simulink model "iiwa_IK_FABRIK_ROS (bkp)"  (R2016b)
settings: Solver=FixedStepAuto  StartTime=0.0  StopTime=inf  FixedStep=0.05  RelTol=1e-3
model workspace (MAT data in the model file):
  SL_ROS_VariableLengthArrays_MaxSizes : struct (value not decoded)
libraries: robotlib x7
(part 2 of 2)

== matlab function iiwa_IK_FABRIK_ROS (bkp)/IK/ik_solver ==
  data: Qs output; js_cur_msg input; T input; Qf output; Q2 output; Q3 output; traj_mode output; x_err output; y_err output; z_err output; alpha_err output; betta_err output; gamma_err output; tr_mode input; out_of_trj input boolean; T_ output; R output
% Based on transformation between /iiwa_base_link and /target_frame from tf
% as on error IK problem is solved and corresponding joint angles 
% changes is sent to arm_state topic

function [Qs, Qf, Q2, Q3, traj_mode, x_err, y_err, z_err, alpha_err,... 
          betta_err, gamma_err, T_, R] = fcn(js_cur_msg, T, tr_mode, out_of_trj)
      
persistent points;
if isempty(points)
    points = zeros(7,3);
    
end

persistent on_traj;
if isempty(on_traj)
    on_traj = true;
end

persistent out_of_;
if isempty(out_of_)
    out_of_ = true;
end

persistent seq;
if isempty(seq)
    seq = 0;
end

persistent x;
if isempty(x)
    x = 0;
end

persistent y;
if isempty(y)
    y = 0;
end

persistent z;
if isempty(z)
    z = 0.1;
end

persistent q;
if isempty(q)
    q = [1, 0, 0, 0];
end

T_ = T;

d01 = 0.36;
d23 = 0.42;
d45 = 0.4;
d67 = 0.126;

th1 = js_cur_msg.Position(1);
th2 = js_cur_msg.Position(2);
th3 = js_cur_msg.Position(3);
th4 = js_cur_msg.Position(4);
th5 = js_cur_msg.Position(5);
th6 = js_cur_msg.Position(6);
th7 = js_cur_msg.Position(7);
th_cur = [th1, th2, th3, th4, th5, th6, th7];
Qs = th_cur;

traj_mode = tr_mode;
out_of_ = out_of_trj;

if (out_of_ == true) % another wired shit
    on_traj = false;
end

%if on_traj == false
    x = T(1);
    y = T(2);
    z = T(3);
    q = [T(4), T(5), T(6), T(7)];
%end

H = [cos(th7)*(sin(th6)*(sin(th4)*(sin(th1)*sin(th3) - cos(th1)*cos(th2)*cos(th3)) - cos(th1)*cos(th4)*sin(th2)) - cos(th6)*(cos(th5)*(cos(th4)*(sin(th1)*sin(th3) - cos(th1)*cos(th2)*cos(th3)) + cos(th1)*sin(th2)*sin(th4)) + sin(th5)*(cos(th3)*sin(th1) + cos(th1)*cos(th2)*sin(th3)))) + sin(th7)*(sin(th5)*(cos(th4)*(sin(th1)*sin(th3) - cos(th1)*cos(th2)*cos(th3)) + cos(th1)*sin(th2)*sin(th4)) - cos(th5)*(cos(th3)*sin(th1) + cos(th1)*cos(th2)*sin(th3))), cos(th7)*(sin(th5)*(cos(th4)*(sin(th1)*sin(th3) - cos(th1)*cos(th2)*cos(th3)) + cos(th1)*sin(th2)*sin(th4)) - cos(th5)*(cos(th3)*sin(th1) + cos(th1)*cos(th2)*sin(th3))) - sin(th7)*(sin(th6)*(sin(th4)*(sin(th1)*sin(th3) - cos(th1)*cos(th2)*cos(th3)) - cos(th1)*cos(th4)*sin(th2)) - cos(th6)*(cos(th5)*(cos(th4)*(sin(th1)*sin(th3) - cos(th1)*cos(th2)*cos(th3)) + cos(th1)*sin(th2)*sin(th4)) + sin(th5)*(cos(th3)*sin(th1) + cos(th1)*cos(th2)*sin(th3)))),   cos(th6)*(sin(th4)*(sin(th1)*sin(th3) - cos(th1)*cos(th2)*cos(th3)) - cos(th1)*cos(th4)*sin(th2)) + sin(th6)*(cos(th5)*(cos(th4)*(sin(th1)*sin(th3) - cos(th1)*cos(th2)*cos(th3)) + cos(th1)*sin(th2)*sin(th4)) + sin(th5)*(cos(th3)*sin(th1) + cos(th1)*cos(th2)*sin(th3))),   d67*(cos(th6)*(sin(th4)*(sin(th1)*sin(th3) - cos(th1)*cos(th2)*cos(th3)) - cos(th1)*cos(th4)*sin(th2)) + sin(th6)*(cos(th5)*(cos(th4)*(sin(th1)*sin(th3) - cos(th1)*cos(th2)*cos(th3)) + cos(th1)*sin(th2)*sin(th4)) + sin(th5)*(cos(th3)*sin(th1) + cos(th1)*cos(th2)*sin(th3)))) + d45*(sin(th4)*(sin(th1)*sin(th3) - cos(th1)*cos(th2)*cos(th3)) - cos(th1)*cos(th4)*sin(th2)) - d23*cos(th1)*sin(th2);...
     -cos(th7)*(sin(th6)*(sin(th4)*(cos(th1)*sin(th3) + cos(th2)*cos(th3)*sin(th1)) + cos(th4)*sin(th1)*sin(th2)) - cos(th6)*(cos(th5)*(cos(th4)*(cos(th1)*sin(th3) + cos(th2)*cos(th3)*sin(th1)) - sin(th1)*sin(th2)*sin(th4)) + sin(th5)*(cos(th1)*cos(th3) - cos(th2)*sin(th1)*sin(th3)))) - sin(th7)*(sin(th5)*(cos(th4)*(cos(th1)*sin(th3) + cos(th2)*cos(th3)*sin(th1)) - sin(th1)*sin(th2)*sin(th4)) - cos(th5)*(cos(th1)*cos(th3) - cos(th2)*sin(th1)*sin(th3))), sin(th7)*(sin(th6)*(sin(th4)*(cos(th1)*sin(th3) + cos(th2)*cos(th3)*sin(th1)) + cos(th4)*sin(th1)*sin(th2)) - cos(th6)*(cos(th5)*(cos(th4)*(cos(th1)*sin(th3) + cos(th2)*cos(th3)*sin(th1)) - sin(th1)*sin(th2)*sin(th4)) + sin(th5)*(cos(th1)*cos(th3) - cos(th2)*sin(th1)*sin(th3)))) - cos(th7)*(sin(th5)*(cos(th4)*(cos(th1)*sin(th3) + cos(th2)*cos(th3)*sin(th1)) - sin(th1)*sin(th2)*sin(th4)) - cos(th5)*(cos(th1)*cos(th3) - cos(th2)*sin(th1)*sin(th3))), - cos(th6)*(sin(th4)*(cos(th1)*sin(th3) + cos(th2)*cos(th3)*sin(th1)) + cos(th4)*sin(th1)*sin(th2)) - sin(th6)*(cos(th5)*(cos(th4)*(cos(th1)*sin(th3) + cos(th2)*cos(th3)*sin(th1)) - sin(th1)*sin(th2)*sin(th4)) + sin(th5)*(cos(th1)*cos(th3) - cos(th2)*sin(th1)*sin(th3))), - d67*(cos(th6)*(sin(th4)*(cos(th1)*sin(th3) + cos(th2)*cos(th3)*sin(th1)) + cos(th4)*sin(th1)*sin(th2)) + sin(th6)*(cos(th5)*(cos(th4)*(cos(th1)*sin(th3) + cos(th2)*cos(th3)*sin(th1)) - sin(th1)*sin(th2)*sin(th4)) + sin(th5)*(cos(th1)*cos(th3) - cos(th2)*sin(th1)*sin(th3)))) - d45*(sin(th4)*(cos(th1)*sin(th3) + cos(th2)*cos(th3)*sin(th1)) + cos(th4)*sin(th1)*sin(th2)) - d23*sin(th1)*sin(th2);...
     cos(th7)*(cos(th6)*(cos(th5)*(cos(th2)*sin(th4) + cos(th3)*cos(th4)*sin(th2)) - sin(th2)*sin(th3)*sin(th5)) + sin(th6)*(cos(th2)*cos(th4) - cos(th3)*sin(th2)*sin(th4))) - sin(th7)*(sin(th5)*(cos(th2)*sin(th4) + cos(th3)*cos(th4)*sin(th2)) + cos(th5)*sin(th2)*sin(th3)),                                                                                                                                                                                     - cos(th7)*(sin(th5)*(cos(th2)*sin(th4) + cos(th3)*cos(th4)*sin(th2)) + cos(th5)*sin(th2)*sin(th3)) - sin(th7)*(cos(th6)*(cos(th5)*(cos(th2)*sin(th4) + cos(th3)*cos(th4)*sin(th2)) - sin(th2)*sin(th3)*sin(th5)) + sin(th6)*(cos(th2)*cos(th4) - cos(th3)*sin(th2)*sin(th4))),                                                                                                                  cos(th6)*(cos(th2)*cos(th4) - cos(th3)*sin(th2)*sin(th4)) - sin(th6)*(cos(th5)*(cos(th2)*sin(th4) + cos(th3)*cos(th4)*sin(th2)) - sin(th2)*sin(th3)*sin(th5)),                                                                                                                                                             d01 + d45*(cos(th2)*cos(th4) - cos(th3)*sin(th2)*sin(th4)) - d67*(sin(th6)*(cos(th5)*(cos(th2)*sin(th4) + cos(th3)*cos(th4)*sin(th2)) - sin(th2)*sin(th3)*sin(th5)) - cos(th6)*(cos(th2)*cos(th4) - cos(th3)*sin(th2)*sin(th4))) + d23*cos(th2);...
                                                                                                                                                                                                                                                                                                                                                                                                                                                                        0,                                                                                                                                                                                                                                                                                                                                                                                                                                                                  0,                                                                                                                                                                                                                                                                              0,                                                                                                                                                                                                                                                                                                                                                                                                           1];  
x_cur = H(1,4);
y_cur = H(2,4);
z_cur = H(3,4);
eul_cur = rotm2eul(H(1:3,1:3));

eul = quat2eul(q);

x_err = x - x_cur;
y_err = y - y_cur;
z_err = z - z_cur;
eul_err = eul - eul_cur;
alpha_err = eul_err(3);
betta_err = eul_err(2);
gamma_err = eul_err(1);
R = [0, 0, 0];

if (on_traj == true)
    Qf = th_cur;
    Q2 = th_cur;
    Q3 = th_cur;
else
    [Qf, R] = IK_FABRIK(x, y, z, q, th_cur); %final pose

    if (tr_mode == true)
        L=1/3;
        x_p2 = (1-L)*x_cur + L*x;
        y_p2 = (1-L)*y_cur + L*y;
        z_p2 = (1-L)*z_cur + L*z;

        Q2 = IK_calc2(x_p2, y_p2, z_p2, q, th_cur); % second pose

        L=2/3;
        x_p3 = (1-L)*x_cur + L*x;
        y_p3 = (1-L)*y_cur + L*y;
        z_p3 = (1-L)*z_cur + L*z;

        Q3 = IK_calc2(x_p3, y_p3, z_p3, q, th_cur); % third pose
        on_traj = true;
    else
        Q2 = Qf;
        Q3 = Qf;
    end
end

seq = seq + 1;
end

function [th_new, deb] = IK_FABRIK(x, y, z, q, th_cur)

p07t = [x; y; z];

d01 = 0.36;
d23 = 0.42;
d45 = 0.4;
d67 = 0.126;

th1 = th_cur(1);
th2 = th_cur(2);
th3 = th_cur(3);
th4 = th_cur(4);
th5 = th_cur(5);
th6 = th_cur(6);
th7 = th_cur(7);

H07 = [[   cos(th7)*(sin(th6)*(sin(th4)*(sin(th1)*sin(th3) - cos(th1)*cos(th2)*cos(th3)) - cos(th1)*cos(th4)*sin(th2)) - cos(th6)*(cos(th5)*(cos(th4)*(sin(th1)*sin(th3) - cos(th1)*cos(th2)*cos(th3)) + cos(th1)*sin(th2)*sin(th4)) + sin(th5)*(cos(th3)*sin(th1) + cos(th1)*cos(th2)*sin(th3)))) + sin(th7)*(sin(th5)*(cos(th4)*(sin(th1)*sin(th3) - cos(th1)*cos(th2)*cos(th3)) + cos(th1)*sin(th2)*sin(th4)) - cos(th5)*(cos(th3)*sin(th1) + cos(th1)*cos(th2)*sin(th3))), cos(th7)*(sin(th5)*(cos(th4)*(sin(th1)*sin(th3) - cos(th1)*cos(th2)*cos(th3)) + cos(th1)*sin(th2)*sin(th4)) - cos(th5)*(cos(th3)*sin(th1) + cos(th1)*cos(th2)*sin(th3))) - sin(th7)*(sin(th6)*(sin(th4)*(sin(th1)*sin(th3) - cos(th1)*cos(th2)*cos(th3)) - cos(th1)*cos(th4)*sin(th2)) - cos(th6)*(cos(th5)*(cos(th4)*(sin(th1)*sin(th3) - cos(th1)*cos(th2)*cos(th3)) + cos(th1)*sin(th2)*sin(th4)) + sin(th5)*(cos(th3)*sin(th1) + cos(th1)*cos(th2)*sin(th3)))),   cos(th6)*(sin(th4)*(sin(th1)*sin(th3) - cos(th1)*cos(th2)*cos(th3)) - cos(th1)*cos(th4)*sin(th2)) + sin(th6)*(cos(th5)*(cos(th4)*(sin(th1)*sin(th3) - cos(th1)*cos(th2)*cos(th3)) + cos(th1)*sin(th2)*sin(th4)) + sin(th5)*(cos(th3)*sin(th1) + cos(th1)*cos(th2)*sin(th3))),   d67*(cos(th6)*(sin(th4)*(sin(th1)*sin(th3) - cos(th1)*cos(th2)*cos(th3)) - cos(th1)*cos(th4)*sin(th2)) + sin(th6)*(cos(th5)*(cos(th4)*(sin(th1)*sin(th3) - cos(th1)*cos(th2)*cos(th3)) + cos(th1)*sin(th2)*sin(th4)) + sin(th5)*(cos(th3)*sin(th1) + cos(th1)*cos(th2)*sin(th3)))) + d45*(sin(th4)*(sin(th1)*sin(th3) - cos(th1)*cos(th2)*cos(th3)) - cos(th1)*cos(th4)*sin(th2)) - d23*cos(th1)*sin(th2)]
       [ - cos(th7)*(sin(th6)*(sin(th4)*(cos(th1)*sin(th3) + cos(th2)*cos(th3)*sin(th1)) + cos(th4)*sin(th1)*sin(th2)) - cos(th6)*(cos(th5)*(cos(th4)*(cos(th1)*sin(th3) + cos(th2)*cos(th3)*sin(th1)) - sin(th1)*sin(th2)*sin(th4)) + sin(th5)*(cos(th1)*cos(th3) - cos(th2)*sin(th1)*sin(th3)))) - sin(th7)*(sin(th5)*(cos(th4)*(cos(th1)*sin(th3) + cos(th2)*cos(th3)*sin(th1)) - sin(th1)*sin(th2)*sin(th4)) - cos(th5)*(cos(th1)*cos(th3) - cos(th2)*sin(th1)*sin(th3))), sin(th7)*(sin(th6)*(sin(th4)*(cos(th1)*sin(th3) + cos(th2)*cos(th3)*sin(th1)) + cos(th4)*sin(th1)*sin(th2)) - cos(th6)*(cos(th5)*(cos(th4)*(cos(th1)*sin(th3) + cos(th2)*cos(th3)*sin(th1)) - sin(th1)*sin(th2)*sin(th4)) + sin(th5)*(cos(th1)*cos(th3) - cos(th2)*sin(th1)*sin(th3)))) - cos(th7)*(sin(th5)*(cos(th4)*(cos(th1)*sin(th3) + cos(th2)*cos(th3)*sin(th1)) - sin(th1)*sin(th2)*sin(th4)) - cos(th5)*(cos(th1)*cos(th3) - cos(th2)*sin(th1)*sin(th3))), - cos(th6)*(sin(th4)*(cos(th1)*sin(th3) + cos(th2)*cos(th3)*sin(th1)) + cos(th4)*sin(th1)*sin(th2)) - sin(th6)*(cos(th5)*(cos(th4)*(cos(th1)*sin(th3) + cos(th2)*cos(th3)*sin(th1)) - sin(th1)*sin(th2)*sin(th4)) + sin(th5)*(cos(th1)*cos(th3) - cos(th2)*sin(th1)*sin(th3))), - d67*(cos(th6)*(sin(th4)*(cos(th1)*sin(th3) + cos(th2)*cos(th3)*sin(th1)) + cos(th4)*sin(th1)*sin(th2)) + sin(th6)*(cos(th5)*(cos(th4)*(cos(th1)*sin(th3) + cos(th2)*cos(th3)*sin(th1)) - sin(th1)*sin(th2)*sin(th4)) + sin(th5)*(cos(th1)*cos(th3) - cos(th2)*sin(th1)*sin(th3)))) - d45*(sin(th4)*(cos(th1)*sin(th3) + cos(th2)*cos(th3)*sin(th1)) + cos(th4)*sin(th1)*sin(th2)) - d23*sin(th1)*sin(th2)]
       [                                                                                                                                                                                         cos(th7)*(cos(th6)*(cos(th5)*(cos(th2)*sin(th4) + cos(th3)*cos(th4)*sin(th2)) - sin(th2)*sin(th3)*sin(th5)) + sin(th6)*(cos(th2)*cos(th4) - cos(th3)*sin(th2)*sin(th4))) - sin(th7)*(sin(th5)*(cos(th2)*sin(th4) + cos(th3)*cos(th4)*sin(th2)) + cos(th5)*sin(th2)*sin(th3)),                                                                                                                                                                                     - cos(th7)*(sin(th5)*(cos(th2)*sin(th4) + cos(th3)*cos(th4)*sin(th2)) + cos(th5)*sin(th2)*sin(th3)) - sin(th7)*(cos(th6)*(cos(th5)*(cos(th2)*sin(th4) + cos(th3)*cos(th4)*sin(th2)) - sin(th2)*sin(th3)*sin(th5)) + sin(th6)*(cos(th2)*cos(th4) - cos(th3)*sin(th2)*sin(th4))),                                                                                                                  cos(th6)*(cos(th2)*cos(th4) - cos(th3)*sin(th2)*sin(th4)) - sin(th6)*(cos(th5)*(cos(th2)*sin(th4) + cos(th3)*cos(th4)*sin(th2)) - sin(th2)*sin(th3)*sin(th5)),                                                                                                                                                             d01 + d45*(cos(th2)*cos(th4) - cos(th3)*sin(th2)*sin(th4)) - d67*(sin(th6)*(cos(th5)*(cos(th2)*sin(th4) + cos(th3)*cos(th4)*sin(th2)) - sin(th2)*sin(th3)*sin(th5)) - cos(th6)*(cos(th2)*cos(th4) - cos(th3)*sin(th2)*sin(th4))) + d23*cos(th2)]
       [                                                                                                                                                                                                                                                                                                                                                                                                                                                                    0,                                                                                                                                                                                                                                                                                                                                                                                                                                                                  0,                                                                                                                                                                                                                                                                              0,                                                                                                                                                                                                                                                                                                                                                                                                           1]];
p07 = H07(1:3,4);
% x07 = H07(1,4);
% y07 = H07(2,4);
% z07 = H07(3,4);

R07 = H07(1:3,1:3);
eul07 = rotm2eul(R07);
eul07t = quat2eul(q);
R07t = quat2rotm(q);

H06 = [[ sin(th6)*(sin(th4)*(sin(th1)*sin(th3) - cos(th1)*cos(th2)*cos(th3)) - cos(th1)*cos(th4)*sin(th2)) - cos(th6)*(cos(th5)*(cos(th4)*(sin(th1)*sin(th3) - cos(th1)*cos(th2)*cos(th3)) + cos(th1)*sin(th2)*sin(th4)) + sin(th5)*(cos(th3)*sin(th1) + cos(th1)*cos(th2)*sin(th3))), sin(th5)*(cos(th4)*(sin(th1)*sin(th3) - cos(th1)*cos(th2)*cos(th3)) + cos(th1)*sin(th2)*sin(th4)) - cos(th5)*(cos(th3)*sin(th1) + cos(th1)*cos(th2)*sin(th3)),   cos(th6)*(sin(th4)*(sin(th1)*sin(th3) - cos(th1)*cos(th2)*cos(th3)) - cos(th1)*cos(th4)*sin(th2)) + sin(th6)*(cos(th5)*(cos(th4)*(sin(th1)*sin(th3) - cos(th1)*cos(th2)*cos(th3)) + cos(th1)*sin(th2)*sin(th4)) + sin(th5)*(cos(th3)*sin(th1) + cos(th1)*cos(th2)*sin(th3))),   d45*(sin(th4)*(sin(th1)*sin(th3) - cos(th1)*cos(th2)*cos(th3)) - cos(th1)*cos(th4)*sin(th2)) - d23*cos(th1)*sin(th2)]
       [ cos(th6)*(cos(th5)*(cos(th4)*(cos(th1)*sin(th3) + cos(th2)*cos(th3)*sin(th1)) - sin(th1)*sin(th2)*sin(th4)) + sin(th5)*(cos(th1)*cos(th3) - cos(th2)*sin(th1)*sin(th3))) - sin(th6)*(sin(th4)*(cos(th1)*sin(th3) + cos(th2)*cos(th3)*sin(th1)) + cos(th4)*sin(th1)*sin(th2)), cos(th5)*(cos(th1)*cos(th3) - cos(th2)*sin(th1)*sin(th3)) - sin(th5)*(cos(th4)*(cos(th1)*sin(th3) + cos(th2)*cos(th3)*sin(th1)) - sin(th1)*sin(th2)*sin(th4)), - cos(th6)*(sin(th4)*(cos(th1)*sin(th3) + cos(th2)*cos(th3)*sin(th1)) + cos(th4)*sin(th1)*sin(th2)) - sin(th6)*(cos(th5)*(cos(th4)*(cos(th1)*sin(th3) + cos(th2)*cos(th3)*sin(th1)) - sin(th1)*sin(th2)*sin(th4)) + sin(th5)*(cos(th1)*cos(th3) - cos(th2)*sin(th1)*sin(th3))), - d45*(sin(th4)*(cos(th1)*sin(th3) + cos(th2)*cos(th3)*sin(th1)) + cos(th4)*sin(th1)*sin(th2)) - d23*sin(th1)*sin(th2)]
       [                                                                                                                cos(th6)*(cos(th5)*(cos(th2)*sin(th4) + cos(th3)*cos(th4)*sin(th2)) - sin(th2)*sin(th3)*sin(th5)) + sin(th6)*(cos(th2)*cos(th4) - cos(th3)*sin(th2)*sin(th4)),                                                                      - sin(th5)*(cos(th2)*sin(th4) + cos(th3)*cos(th4)*sin(th2)) - cos(th5)*sin(th2)*sin(th3),                                                                                                                  cos(th6)*(cos(th2)*cos(th4) - cos(th3)*sin(th2)*sin(th4)) - sin(th6)*(cos(th5)*(cos(th2)*sin(th4) + cos(th3)*cos(th4)*sin(th2)) - sin(th2)*sin(th3)*sin(th5)),                                              d01 + d45*(cos(th2)*cos(th4) - cos(th3)*sin(th2)*sin(th4)) + d23*cos(th2)]
       [                                                                                                                                                                                                                                                                            0,                                                                                                                                                             0,                                                                                                                                                                                                                                                                              0,                                                                                                                      1]];

R06 = H06(1:3,1:3);
p06 = H06(1:3,4);
p06t = p07t - d67*R07t*[0;0;1];

deb = [0, 0, 0];

if (abs(norm(p07) - norm(p07t))<0.01)
   if (abs(norm(p06) - norm(p06t))<0.01)
       R7t_7 = transpose(R06)*R07t;
       deb = rotm2eul(R7t_7);
       th7 = deb(1);%-atan2(R7t_7(2,1),R7t_7(1,1));
   end
end

% if (H(2,1) == 0 && H(1,1) == 0)
%     yaw7 = 0;
% yaw7 = ;
% [yaw7t, pitch7t, roll7t] = quat2angle(q);

% H01 = [[ cos(th1), 0,  sin(th1),   0]
%        [ sin(th1), 0, -cos(th1),   0]
%        [        0, 1,         0, d01]
%        [        0, 0,         0,   1]];
%    
% H02 = [[ cos(th1)*cos(th2), -sin(th1), -cos(th1)*sin(th2),   0]
%        [ cos(th2)*sin(th1),  cos(th1), -sin(th1)*sin(th2),   0]
%        [          sin(th2),         0,           cos(th2), d01]
%        [                 0,         0,                  0,   1]];
%    
% H03 = [[ cos(th1)*cos(th2)*cos(th3) - sin(th1)*sin(th3), -cos(th1)*sin(th2), cos(th3)*sin(th1) + cos(th1)*cos(th2)*sin(th3), -d23*cos(th1)*sin(th2)]
%        [ cos(th1)*sin(th3) + cos(th2)*cos(th3)*sin(th1), -sin(th1)*sin(th2), cos(th2)*sin(th1)*sin(th3) - cos(th1)*cos(th3), -d23*sin(th1)*sin(th2)]
%        [                              cos(th3)*sin(th2),           cos(th2),                              sin(th2)*sin(th3),     d01 + d23*cos(th2)]
%        [                                              0,                  0,                                              0,                      1]];
% 
% H04 = [[ - cos(th4)*(sin(th1)*sin(th3) - cos(th1)*cos(th2)*cos(th3)) - cos(th1)*sin(th2)*sin(th4), - cos(th3)*sin(th1) - cos(th1)*cos(th2)*sin(th3),   sin(th4)*(sin(th1)*sin(th3) - cos(th1)*cos(th2)*cos(th3)) - cos(th1)*cos(th4)*sin(th2), -d23*cos(th1)*sin(th2)]
%        [   cos(th4)*(cos(th1)*sin(th3) + cos(th2)*cos(th3)*sin(th1)) - sin(th1)*sin(th2)*sin(th4),   cos(th1)*cos(th3) - cos(th2)*sin(th1)*sin(th3), - sin(th4)*(cos(th1)*sin(th3) + cos(th2)*cos(th3)*sin(th1)) - cos(th4)*sin(th1)*sin(th2), -d23*sin(th1)*sin(th2)]
%        [                                           cos(th2)*sin(th4) + cos(th3)*cos(th4)*sin(th2),                               -sin(th2)*sin(th3),                                           cos(th2)*cos(th4) - cos(th3)*sin(th2)*sin(th4),     d01 + d23*cos(th2)]
%        [                                                                                        0,                                                0,                                                                                        0,                      1]];
% 
% H05 = [[ - cos(th5)*(cos(th4)*(sin(th1)*sin(th3) - cos(th1)*cos(th2)*cos(th3)) + cos(th1)*sin(th2)*sin(th4)) - sin(th5)*(cos(th3)*sin(th1) + cos(th1)*cos(th2)*sin(th3)),   sin(th4)*(sin(th1)*sin(th3) - cos(th1)*cos(th2)*cos(th3)) - cos(th1)*cos(th4)*sin(th2), cos(th5)*(cos(th3)*sin(th1) + cos(th1)*cos(th2)*sin(th3)) - sin(th5)*(cos(th4)*(sin(th1)*sin(th3) - cos(th1)*cos(th2)*cos(th3)) + cos(th1)*sin(th2)*sin(th4)),   d45*(sin(th4)*(sin(th1)*sin(th3) - cos(th1)*cos(th2)*cos(th3)) - cos(th1)*cos(th4)*sin(th2)) - d23*cos(th1)*sin(th2)]
%        [   cos(th5)*(cos(th4)*(cos(th1)*sin(th3) + cos(th2)*cos(th3)*sin(th1)) - sin(th1)*sin(th2)*sin(th4)) + sin(th5)*(cos(th1)*cos(th3) - cos(th2)*sin(th1)*sin(th3)), - sin(th4)*(cos(th1)*sin(th3) + cos(th2)*cos(th3)*sin(th1)) - cos(th4)*sin(th1)*sin(th2), sin(th5)*(cos(th4)*(cos(th1)*sin(th3) + cos(th2)*cos(th3)*sin(th1)) - sin(th1)*sin(th2)*sin(th4)) - cos(th5)*(cos(th1)*cos(th3) - cos(th2)*sin(th1)*sin(th3)), - d45*(sin(th4)*(cos(th1)*sin(th3) + cos(th2)*cos(th3)*sin(th1)) + cos(th4)*sin(th1)*sin(th2)) - d23*sin(th1)*sin(th2)]
%        [                                                                          cos(th5)*(cos(th2)*sin(th4) + cos(th3)*cos(th4)*sin(th2)) - sin(th2)*sin(th3)*sin(th5),                                           cos(th2)*cos(th4) - cos(th3)*sin(th2)*sin(th4),                                                                        sin(th5)*(cos(th2)*sin(th4) + cos(th3)*cos(th4)*sin(th2)) + cos(th5)*sin(th2)*sin(th3),                                              d01 + d45*(cos(th2)*cos(th4) - cos(th3)*sin(th2)*sin(th4)) + d23*cos(th2)]
%        [                                                                                                                                                               0,                                                                                        0,                                                                                                                                                             0,                                                                                                                      1]];
% 
% H06 = [[ sin(th6)*(sin(th4)*(sin(th1)*sin(th3) - cos(th1)*cos(th2)*cos(th3)) - cos(th1)*cos(th4)*sin(th2)) - cos(th6)*(cos(th5)*(cos(th4)*(sin(th1)*sin(th3) - cos(th1)*cos(th2)*cos(th3)) + cos(th1)*sin(th2)*sin(th4)) + sin(th5)*(cos(th3)*sin(th1) + cos(th1)*cos(th2)*sin(th3))), sin(th5)*(cos(th4)*(sin(th1)*sin(th3) - cos(th1)*cos(th2)*cos(th3)) + cos(th1)*sin(th2)*sin(th4)) - cos(th5)*(cos(th3)*sin(th1) + cos(th1)*cos(th2)*sin(th3)),   cos(th6)*(sin(th4)*(sin(th1)*sin(th3) - cos(th1)*cos(th2)*cos(th3)) - cos(th1)*cos(th4)*sin(th2)) + sin(th6)*(cos(th5)*(cos(th4)*(sin(th1)*sin(th3) - cos(th1)*cos(th2)*cos(th3)) + cos(th1)*sin(th2)*sin(th4)) + sin(th5)*(cos(th3)*sin(th1) + cos(th1)*cos(th2)*sin(th3))),   d45*(sin(th4)*(sin(th1)*sin(th3) - cos(th1)*cos(th2)*cos(th3)) - cos(th1)*cos(th4)*sin(th2)) - d23*cos(th1)*sin(th2)]
%        [ cos(th6)*(cos(th5)*(cos(th4)*(cos(th1)*sin(th3) + cos(th2)*cos(th3)*sin(th1)) - sin(th1)*sin(th2)*sin(th4)) + sin(th5)*(cos(th1)*cos(th3) - cos(th2)*sin(th1)*sin(th3))) - sin(th6)*(sin(th4)*(cos(th1)*sin(th3) + cos(th2)*cos(th3)*sin(th1)) + cos(th4)*sin(th1)*sin(th2)), cos(th5)*(cos(th1)*cos(th3) - cos(th2)*sin(th1)*sin(th3)) - sin(th5)*(cos(th4)*(cos(th1)*sin(th3) + cos(th2)*cos(th3)*sin(th1)) - sin(th1)*sin(th2)*sin(th4)), - cos(th6)*(sin(th4)*(cos(th1)*sin(th3) + cos(th2)*cos(th3)*sin(th1)) + cos(th4)*sin(th1)*sin(th2)) - sin(th6)*(cos(th5)*(cos(th4)*(cos(th1)*sin(th3) + cos(th2)*cos(th3)*sin(th1)) - sin(th1)*sin(th2)*sin(th4)) + sin(th5)*(cos(th1)*cos(th3) - cos(th2)*sin(th1)*sin(th3))), - d45*(sin(th4)*(cos(th1)*sin(th3) + cos(th2)*cos(th3)*sin(th1)) + cos(th4)*sin(th1)*sin(th2)) - d23*sin(th1)*sin(th2)]
%        [                                                                                                                cos(th6)*(cos(th5)*(cos(th2)*sin(th4) + cos(th3)*cos(th4)*sin(th2)) - sin(th2)*sin(th3)*sin(th5)) + sin(th6)*(cos(th2)*cos(th4) - cos(th3)*sin(th2)*sin(th4)),                                                                      - sin(th5)*(cos(th2)*sin(th4) + cos(th3)*cos(th4)*sin(th2)) - cos(th5)*sin(th2)*sin(th3),                                                                                                                  cos(th6)*(cos(th2)*cos(th4) - cos(th3)*sin(th2)*sin(th4)) - sin(th6)*(cos(th5)*(cos(th2)*sin(th4) + cos(th3)*cos(th4)*sin(th2)) - sin(th2)*sin(th3)*sin(th5)),                                              d01 + d45*(cos(th2)*cos(th4) - cos(th3)*sin(th2)*sin(th4)) + d23*cos(th2)]
%        [                                                                                                                                                                                                                                                                            0,                                                                                                                                                             0,                                                                                                                                                                                                                                                                              0,                                                                                                                      1]];
% 
% 
% x01 = H01(1,4);
% y01 = H01(2,4);
% z01 = H01(3,4);
% x02 = H02(1,4);
% y02 = H02(2,4);
% z02 = H02(3,4);
% x03 = H03(1,4);
% y03 = H03(2,4);
% z03 = H03(3,4);
% x04 = H04(1,4);
% y04 = H04(2,4);
% z04 = H04(3,4);
% x05 = H05(1,4);
% y05 = H05(2,4);
% z05 = H05(3,4);
% x06 = H06(1,4);
% y06 = H06(2,4);
% z06 = H06(3,4);
% x07 = H07(1,4);
% y07 = H07(2,4);
% z07 = H07(3,4);
%eul_cur = rotm2eul(H(1:3,1:3));
%eul = quat2eul(q);



th_new = [th1, th2, th3, th4, th5, th6, th7];
end

function [th_new] = IK_calc(x, y, z, q, th_cur)
th1 = th_cur(1);
th2 = th_cur(2);
th3 = th_cur(3);
th4 = th_cur(4);
th5 = th_cur(5);
th6 = th_cur(6);
th7 = th_cur(7);

d01 = 0.36;
d23 = 0.42;
d45 = 0.4;
d67 = 0.126;

R0T = quat2rotm(q);
p0T = [x; y; z];
p05 = p0T - d67*R0T*[0;0;1];

% th1

th1_1 = 0;
th1_2 = 0;

k1 = 0; %shows whether +pi is used or not
if (p05(1) ~= 0) && (p05(2) ~= 0)
    th1_1 = atan2(p05(2), p05(1));
    if th1_1 > 0
        th1_2 = th1_1 - pi;
    else %th <= 0
        th1_2 = th1_1 + pi;
    end
    if sign(th1) == sign(th1_1)
        if (abs(th1 - th1_1) <= abs(th1 - th1_2))
            th1 = th1_1;
        else
            th1 = th1_2;
        end
    else
        if (abs(abs(th1) - abs(th1_1)) <= abs(abs(th1) - abs(th1_2)))
            th1 = th1_1;
        else
            th1 = th1_2;
            
        end
    end
end

c = sqrt(p05(1)^2 + p05(2)^2);
b = p05(3) - sign(p05(3))*d01;
a = sqrt(b^2 + c^2);

% th4
if sqrt(p05(1)^2 + p05(2)^2 + (abs(p05(3))-d01)^2) >= (d23 + d45)
    th4 = 0;
else
    cth4 = (b^2 + c^2 - (d23)^2 - (d45)^2)/(2*d23*d45);
    th4_1 = atan2((sqrt(1-(cth4)^2)), cth4);
    th4_2 = atan2(-(sqrt(1-(cth4)^2)), cth4);
    if (abs(th4 - th4_1) <= abs(th4 - th4_2))
            th4 = th4_1;
    else
            th4 = th4_2;
    end
end

% th2
th2_1 = atan2(b,c) - atan2(d45*sin(th4),d23+d45*cos(th4))-pi/2;
th2 = th2_1;

th3 = 0;    %fixed

% th5
R03 = [[ cos(th1)*cos(th2)*cos(th4) - cos(th1)*sin(th2)*sin(th4), -sin(th1), - cos(th1)*cos(th2)*sin(th4) - cos(th1)*cos(th4)*sin(th2)];...
       [ cos(th2)*cos(th4)*sin(th1) - sin(th1)*sin(th2)*sin(th4),  cos(th1), - cos(th2)*sin(th1)*sin(th4) - cos(th4)*sin(th1)*sin(th2)];...
       [                   cos(th2)*sin(th4) + cos(th4)*sin(th2),         0,                     cos(th2)*cos(th4) - sin(th2)*sin(th4)]];


R36 = transpose(R03)*R0T;   
th6 = atan2(sqrt(1-R36(3,3)^2),R36(3,3));

th5 = atan2(-R36(2,3),-R36(1,3));

th7 = atan2(-R36(3,2),R36(3,1));

th_new = [th1, th2, th3, th4, th5, th6, th7];

end


function [th_new] = IK_calc2(x, y, z, q, th_cur)
th1 = th_cur(1);
th2 = th_cur(2);
th3 = th_cur(3);
th4 = th_cur(4);
th5 = th_cur(5);
th6 = th_cur(6);
th7 = th_cur(7);

d01 = 0.36;
d23 = 0.42;
d45 = 0.4;
d67 = 0.126;

R0T = quat2rotm(q);
p0T = [x; y; z];
p05 = p0T - d67*R0T*[0;0;1];

% th1
if (p05(1) ~= 0) && (p05(2) ~= 0)
    th1 = atan2(p05(2), p05(1));
    c = sqrt(p05(1)^2 + p05(2)^2);
else
    c = 0;
end

b = p05(3) - sign(p05(3))*d01;

if (p05(3) ~= 0)
    a = sqrt(b^2 + c^2);
else
    a = 0;
end

% th4
if sqrt(p05(1)^2 + p05(2)^2 + (abs(p05(3))-d01)^2) >= (d23 + d45)
    th4 = 0;
else
    cth4 = (b^2 + c^2 - (d23)^2 - (d45)^2)/(2*d23*d45);
    th4_1 = atan2((sqrt(1-(cth4)^2)), cth4);
    th4_2 = atan2(-(sqrt(1-(cth4)^2)), cth4);
    if (abs(th4 - th4_1) <= abs(th4 - th4_2))
            th4 = th4_1;
    else
            th4 = th4_2;
    end
end

% th2
th2 = atan2(b,c) - atan2(d45*sin(th4),d23+d45*cos(th4))-pi/2;

th3 = 0;    %fixed

% th5
R03 = [[ cos(th1)*cos(th2)*cos(th4) - cos(th1)*sin(th2)*sin(th4), -sin(th1), - cos(th1)*cos(th2)*sin(th4) - cos(th1)*cos(th4)*sin(th2)];...
       [ cos(th2)*cos(th4)*sin(th1) - sin(th1)*sin(th2)*sin(th4),  cos(th1), - cos(th2)*sin(th1)*sin(th4) - cos(th4)*sin(th1)*sin(th2)];...
       [                   cos(th2)*sin(th4) + cos(th4)*sin(th2),         0,                     cos(th2)*cos(th4) - sin(th2)*sin(th4)]];


R36 = transpose(R03)*R0T;   
th6 = atan2(sqrt(1-R36(3,3)^2),R36(3,3));

th5 = atan2(-R36(2,3),-R36(1,3));

th7 = atan2(-R36(3,2),R36(3,1));

th_new = [th1, th2, th3, th4, th5, th6, th7];

end

== matlab function iiwa_IK_FABRIK_ROS (bkp)/error_calc ==
  data: tf_in_msg input Bus: SL_Bus_iiwa_IK_FABRIK_ROS_tf2_msgs_TFMessage; T output double; alpha output; betta output; gamma output; x output; y output; z output; q output; tr_mode output
% Based on transformation between /iiwa_base_link and /target_frame from tf
% as on error IK problem is solved and corresponding joint angles 
% changes is sent to arm_state topic

function [T, alpha, betta, gamma, x, y, z, q, tr_mode]  = fcn(tf_in_msg)

% Set it by "true" to turn it on
persistent traj_mode;
if isempty(traj_mode)
    traj_mode = false;
end

persistent x_;
if isempty(x_)
    x_ = 0;
end

persistent y_;
if isempty(y_)
    y_ = 0;
end

persistent z_;
if isempty(z_)
    z_ = 0;
end

persistent q_;
if isempty(q_)
    q_ = [1, 0, 0, 0];
end

persistent alpha_;
if isempty(alpha_)
    alpha_ = 0;
end

persistent betta_;
if isempty(betta_)
    betta_ = 0;
end

persistent gamma_;
if isempty(gamma_)
    gamma_ = 0;
end

persistent roll_;
if isempty(roll_)
    roll_ = 0;
end

persistent pitch_;
if isempty(pitch_)
    pitch_ = 0;
end

persistent yaw_;
if isempty(yaw_)
    yaw_ = 0;
end

tf_n = tf_in_msg.Transforms_SL_Info.CurrentLength;

%%%%%%%%%%%%%%%%%%%%%%%%%%%%%%%%%%%%%%%%%%%%%%%%
par = 'iiwa_base_link';
ch1 = 'tool_target';

x = 0.0; 
y = 0.0; 
z = 0.0; 
q = [1, 0, 0, 0];
alpha = 0.0; 
betta = 0.0; 
gamma = 0.0;

%for i=1:tf_n
if (tf_n==1)
    i=1;
    child_fr = tf_in_msg.Transforms(i).ChildFrameId;
    parent_fr = tf_in_msg.Transforms(i).Header.FrameId;
    if (strncmp(char(parent_fr), par, length(par)))
       if (strncmp(char(child_fr), ch1, length(ch1)))
           x = tf_in_msg.Transforms(i).Transform.Translation.X;
           y = tf_in_msg.Transforms(i).Transform.Translation.Y;
           z = tf_in_msg.Transforms(i).Transform.Translation.Z;
           q = [tf_in_msg.Transforms(i).Transform.Rotation.W,...
                tf_in_msg.Transforms(i).Transform.Rotation.X,...
                tf_in_msg.Transforms(i).Transform.Rotation.Y,...
                tf_in_msg.Transforms(i).Transform.Rotation.Z];
           eul = quat2eul(q);
           %[yaw, pitch, roll] = quat2angle(q);
           alpha = eul(3);
           betta = eul(2);
           gamma = eul(1);
           x_ = x; y_ = y; z_ = z; q_ = q;
           alpha_ = alpha; betta_ = betta; gamma_ = gamma;
           %yaw_ = yaw; pitch_ = pitch; roll_ = roll;
       end
    end
end

tr_mode = traj_mode;

T = double([x_,y_,z_,q_, alpha_, betta_, gamma_]);
end
